simulink model "mfordmodel_v1"  (R2023a)
settings: Solver=ode45  StartTime=0.0  StopTime=10.0  RelTol=1e-3  EnableMultiTasking=on
undefined symbols (not defined in the file): ABV_RATIO_SW, AC_OFF_DLY, ACLOD, AUTO_TRNS_SW, BRAKE_DNDT_X, BZZRPM, BZZRPM_ALT, BZZTM, BZZTM_ALT, CMD_LITOFF, CMD_STABLE, CO_ST_ECT__A, COOL_BASE, DAS_BKDLY_A, DAS_CNT, DAS_CTDLY, DAS_LC_SW__A, DASCLP_5INH, DASCTL, DASMHYST, DASMPH, DEBYCP, DES_BASE, DPNEU_MUL, DSDRPM_DN_TC, DSDRPM_OFF, DSDRPM_UP_TC, EDF_DELAY, EDFHP, ETC_CL_TP, ETC_HP, GR_CM_CREEP, HCAM_ACT_CLP, HEDFHP, HEDFRPM, HICAM_PS, IAC_CAL_SW, IAC_ER_TM1, IAC_ER_TM2, IAC_ER_TM4, IAC_HI_LIM__A, IAC_ISFL_OBD, IAC_KAM_SW, IAC_LO_LIM__A, IAC_MON_TM, IAC_OT_REQ, IAC_RUN_TM, IAC_TP_OBD, IAC_TR_DAS, IAC_TST_DC, ID_DAS__A, ID_NOVS__A, IDVS_CH__A, IDVS_SL__A, IPSI_SW, IPSIDLY, IS_DRBASE__A, IS_DRBASE_A__A, IS_NUBASE__A, IS_NUBASE_A__A ... (+35)
libraries: simulink x2
(part 8 of 12)

== system mfordmodel_v1/iac_v04_001_001/normal_mode/iscflg_module/idle_rpm_controller/iscpsi_calc ==
  ml_tc_sw : Inport
  ml_iscpsi_sw : Inport  Port=2
  desmaf_pre : Inport  Port=3
  dsdrpm : Inport  Port=4
  rpmerr_a : Inport  Port=5
  iac_dlt_time : Inport  Port=6
  do_iscpsi_calc : TriggerPort  TriggerType=function-call  VariantControl=(inherit)
  Constant : Constant  Value=0.0
  Multiport Switch : MultiPortSwitch  Inputs=2
  Multiport Switch1 : MultiPortSwitch  Inputs=2
  Product : Product  Inputs=3  InputSameDT=on  RndMeth=Zero  SaturateOnIntegerOverflow=on  OutDataTypeStr=Inherit: Same as first input
  Product1 : Product  Inputs=*/  InputSameDT=on  RndMeth=Zero  SaturateOnIntegerOverflow=on  OutDataTypeStr=Inherit: Same as first input
  Product2 : Product  Inputs=*/  InputSameDT=on  RndMeth=Zero  SaturateOnIntegerOverflow=on  OutDataTypeStr=Inherit: Same as first input
  TC_OVER : Subsystem  mask(Constant){constant=TC_OVER}
      mask help: Constant Block. Will dispaly constant name and value on the icon of the block
      mask init:
      | if isletter(constant(1))
      |   const = evalin('base',constant);
      |   name = constant;
      | else
      |   const = str2num(constant);
      |   name = 'CONST';
      | end;
      mask Display: fprintf('%s = %.4f',name,const);
  TC_UNDER : Subsystem  mask(Constant){constant=TC_UNDER}
      mask help: Constant Block. Will dispaly constant name and value on the icon of the block
      mask init:
      | if isletter(constant(1))
      |   const = evalin('base',constant);
      |   name = constant;
      | else
      |   const = str2num(constant);
      |   name = 'CONST';
      | end;
      mask Display: fprintf('%s = %.4f',name,const);
  iscpsi : Outport
  wires:
  iac_dlt_time/1 -> Product2/1
  ml_tc_sw/1 -> Multiport Switch/1
  TC_OVER/1(Out) -> Multiport Switch/2
  TC_UNDER/1(Out) -> Multiport Switch/3
  Constant/1 -> Multiport Switch1/3
  ml_iscpsi_sw/1 -> Multiport Switch1/1
  Multiport Switch1/1 -> iscpsi/1  "iscpsi"
  Product/1 -> Multiport Switch1/2
  Multiport Switch/1 -> Product2/2
  Product2/1 -> Product/2
  rpmerr_a/1 -> Product/3
  dsdrpm/1 -> Product1/2
  desmaf_pre/1 -> Product1/1
  Product1/1 -> Product/1

== system mfordmodel_v1/iac_v04_001_001/normal_mode/iscflg_module/idle_rpm_controller/rpmerr_calc ==
  dsdrpm : Inport
  engine_speed : Inport  Port=2
  iac_dlt_time : Inport  Port=3
  ml_init_sw : Inport  Port=4
  do_rpmerr_calc : TriggerPort  TriggerType=function-call  VariantControl=(inherit)
  Constant3 : Constant  Value=0.0
  Constant4 : Constant  Value=0.0
  Multiport Switch4 : MultiPortSwitch  Inputs=2
  Multiport Switch5 : MultiPortSwitch  Inputs=2
  ROLAV_TC_DT_in : Subsystem  mask(Rolling Average - Time Constant){TAU=TCBPA}
      mask prompts: TAU "Time Constant"
      mask help: Rolling Average - Time Constant. This filter block is the first order approximation using a time constant. Inputs include the time constant (entered through this dialogue), old_ave which is the previous average value, new_value which is the new filter to filter toward, and the delta_time which is elapsed time over which to perform the filter equation.
      mask init:
      | if isletter(TAU(1))
      |   tc = evalin('base',TAU);
      |   name = TAU;
      | else
      |   tc = str2num(TAU);
      |   name = 'TC';
      | end;
      mask Display: fprintf('%s = %.4f',name,tc);
  Sum2 : Sum  Inputs=+-  InputSameDT=on  SaturateOnIntegerOverflow=on  OutDataTypeStr=Inherit: Same as first input
  Unit Delay : UnitDelay  SampleTime=-1
  rpmerr : Outport
  rpmerr_a : Outport  Port=2
  wires:
  ml_init_sw/1 -> Multiport Switch5/1, Multiport Switch4/1
  Multiport Switch5/1 -> Unit Delay/1, rpmerr_a/1  "rpmerr_a"
  Constant4/1 -> Multiport Switch5/3
  ROLAV_TC_DT_in/1(new_ave) -> Multiport Switch5/2  "rpmerr_a"
  Sum2/1 -> Multiport Switch4/2, ROLAV_TC_DT_in/1(new_value)  "rpmerr"
  Constant3/1 -> Multiport Switch4/3
  Multiport Switch4/1 -> rpmerr/1  "rpmerr"
  iac_dlt_time/1 -> ROLAV_TC_DT_in/3(delta_time)
  Unit Delay/1 -> ROLAV_TC_DT_in/2(old_ave)
  dsdrpm/1 -> Sum2/1
  engine_speed/1 -> Sum2/2

== system mfordmodel_v1/iac_v04_001_001/normal_mode/iscflg_module/iscflg_modes/1 ==
  note: Timer Control calls functions within the Time Calculator
      | after using the flags 'increment_flag' and 'decrement_flag'
      | to determine the direction of the timer.
  note: timer14/TIMER
  trig_time : Inport
  trig_reset : Inport  Port=2
  reset value : Inport  Port=3
  inc flag : Inport  Port=4
  dec flag : Inport  Port=5
  Event Triggers : Mux  Inputs=2
  Time Calculator : Subsystem
  Timer Control : Stateflow chart  TreatAsAtomicUnit=on
  timer : Outport
  wires:
  reset value/1 -> Time Calculator/5(reset_value)  "reset_value"
  trig_reset/1 -> Event Triggers/2  "trig_reset"
  trig_time/1 -> Event Triggers/1  "trig_timer"
  Event Triggers/1 -> Timer Control/Trigger
  Time Calculator/1(timer) -> timer/1  "timer"
  Timer Control/1(count_direction) -> Time Calculator/1(count_direction)  "count_direction"
  Timer Control/2(reset_flag) -> Time Calculator/2(reset_val)  "reset_flag"
  Timer Control/3(do_delta_time()) -> Time Calculator/3(do_delta_time)  "do_delta_time"
  Timer Control/4(do_timer()) -> Time Calculator/4(do_timer)  "do_timer"
  dec flag/1 -> Timer Control/2(decr_flag)  "decrement_flag"
  inc flag/1 -> Timer Control/1(incr_flag)  "increment_flag"

== system mfordmodel_v1/iac_v04_001_001/normal_mode/iscflg_module/iscflg_modes/2 ==
  note: Timer Control calls functions within the Time Calculator
      | after using the flags 'increment_flag' and 'decrement_flag'
      | to determine the direction of the timer.
  note: timer14/TIMER
  trig_time : Inport
  trig_reset : Inport  Port=2
  reset value : Inport  Port=3
  inc flag : Inport  Port=4
  dec flag : Inport  Port=5
  Event Triggers : Mux  Inputs=2
  Time Calculator : Subsystem
  Timer Control : Stateflow chart  TreatAsAtomicUnit=on
  timer : Outport
  wires:
  reset value/1 -> Time Calculator/5(reset_value)  "reset_value"
  trig_reset/1 -> Event Triggers/2  "trig_reset"
  trig_time/1 -> Event Triggers/1  "trig_timer"
  Event Triggers/1 -> Timer Control/Trigger
  Time Calculator/1(timer) -> timer/1  "timer"
  Timer Control/1(count_direction) -> Time Calculator/1(count_direction)  "count_direction"
  Timer Control/2(reset_flag) -> Time Calculator/2(reset_val)  "reset_flag"
  Timer Control/3(do_delta_time()) -> Time Calculator/3(do_delta_time)  "do_delta_time"
  Timer Control/4(do_timer()) -> Time Calculator/4(do_timer)  "do_timer"
  dec flag/1 -> Timer Control/2(decr_flag)  "decrement_flag"
  inc flag/1 -> Timer Control/1(incr_flag)  "increment_flag"

== system mfordmodel_v1/iac_v04_001_001/normal_mode/iscflg_module/preposition/idle_ppm_calc ==
  ml_mul_sw : Inport
  dsdrpm : Inport  Port=2
  engine_speed : Inport  Port=3
  ect : Inport  Port=4
  vspd : Inport  Port=5
  dstpbr : Inport  Port=6
  ratch : Inport  Port=7
  do_idle_ppm_calc : TriggerPort  TriggerType=function-call  VariantControl=(inherit)
  CONSTANT : Subsystem  mask(Constant){constant=DELHYS}
      mask help: Constant Block. Will dispaly constant name and value on the icon of the block
      mask init:
      | if isletter(constant(1))
      |   const = evalin('base',constant);
      |   name = constant;
      | else
      |   const = str2num(constant);
      |   name = 'CONST';
      | end;
      mask Display: fprintf('%s = %.4f',name,const);
  CONSTANT1 : Subsystem  mask(Constant){constant=DMAX_NEU_MOD}
      mask help: Constant Block. Will dispaly constant name and value on the icon of the block
      mask init:
      | if isletter(constant(1))
      |   const = evalin('base',constant);
      |   name = constant;
      | else
      |   const = str2num(constant);
      |   name = 'CONST';
      | end;
      mask Display: fprintf('%s = %.4f',name,const);
  CONSTANT2 : Subsystem  mask(Constant){constant=DASPTK}
      mask help: Constant Block. Will dispaly constant name and value on the icon of the block
      mask init:
      | if isletter(constant(1))
      |   const = evalin('base',constant);
      |   name = constant;
      | else
      |   const = str2num(constant);
      |   name = 'CONST';
      | end;
      mask Display: fprintf('%s = %.4f',name,const);
  Constant1 : Constant  Value=1.0
  Constant2 : Constant  Value=1.99
  Constant3 : Constant  Value=0.0
  FN814 : Subsystem  mask(2-D, piece-wise, linear interpolation){CAL_FUNC=FN814}
      mask prompts: CAL_FUNC "Calibration function name"
      mask help:
      | Performs piece-wise linear interpolation.
      |
      | Output is NOT extrapolated beyond the input range.  If the input value presented to the block lies outside the range specified in the block's parameter, then the value is treated as though it has the value of the nearest value in the range.
      mask init: same as mfordmodel_v1/iac_v04_001_001/activate_desired_rpm/rpm_calcs/lookup_2d
      mask Help:
      | Enter the name of the calibration function.
      | (e.g. EGM_VA_ECT_MULT)
      mask Display:
      | fprintf('%s',CAL_FUNC);
      | plot(calfunc.X,calfunc.Y,max_x*1.05,max_y*1.05,min_x,min_y);
  FN830__A : Subsystem  mask(2-D, piece-wise, linear interpolation){CAL_FUNC=FN830__A}
      mask prompts: CAL_FUNC "Calibration function name"
      mask help:
      | Performs piece-wise linear interpolation.
      |
      | Output is NOT extrapolated beyond the input range.  If the input value presented to the block lies outside the range specified in the block's parameter, then the value is treated as though it has the value of the nearest value in the range.
      mask init: same as mfordmodel_v1/iac_v04_001_001/activate_desired_rpm/rpm_calcs/lookup_2d
      mask Help:
      | Enter the name of the calibration function.
      | (e.g. EGM_VA_ECT_MULT)
      mask Display:
      | fprintf('%s',CAL_FUNC);
      | plot(calfunc.X,calfunc.Y,max_x*1.05,max_y*1.05,min_x,min_y);
  FN882A1 : Subsystem  mask(2-D, piece-wise, linear interpolation){CAL_FUNC=FN882A__A}
      mask prompts: CAL_FUNC "Calibration function name"
      mask help:
      | Performs piece-wise linear interpolation.
      |
      | Output is NOT extrapolated beyond the input range.  If the input value presented to the block lies outside the range specified in the block's parameter, then the value is treated as though it has the value of the nearest value in the range.
      mask init: same as mfordmodel_v1/iac_v04_001_001/activate_desired_rpm/rpm_calcs/lookup_2d
      mask Help:
      | Enter the name of the calibration function.
      | (e.g. EGM_VA_ECT_MULT)
      mask Display:
      | fprintf('%s',CAL_FUNC);
      | plot(calfunc.X,calfunc.Y,max_x*1.05,max_y*1.05,min_x,min_y);
  FN891 : Subsystem  mask(2-D, piece-wise, linear interpolation){CAL_FUNC=FN891}
      mask prompts: CAL_FUNC "Calibration function name"
      mask help:
      | Performs piece-wise linear interpolation.
      |
      | Output is NOT extrapolated beyond the input range.  If the input value presented to the block lies outside the range specified in the block's parameter, then the value is treated as though it has the value of the nearest value in the range.
      mask init: same as mfordmodel_v1/iac_v04_001_001/activate_desired_rpm/rpm_calcs/lookup_2d
      mask Help:
      | Enter the name of the calibration function.
      | (e.g. EGM_VA_ECT_MULT)
      mask Display:
      | fprintf('%s',CAL_FUNC);
      | plot(calfunc.X,calfunc.Y,max_x*1.05,max_y*1.05,min_x,min_y);
  MinMax : MinMax  Inputs=2  InputSameDT=on  SaturateOnIntegerOverflow=on
  MinMax1 : MinMax  Function=max  Inputs=2  InputSameDT=on  SaturateOnIntegerOverflow=on
  MinMax3 : MinMax  Inputs=2  InputSameDT=on  SaturateOnIntegerOverflow=on
  Multiport Switch4 : MultiPortSwitch  Inputs=2
  Product2 : Product  InputSameDT=on  RndMeth=Zero  SaturateOnIntegerOverflow=on  OutDataTypeStr=Inherit: Same as first input
  Product4 : Product  Inputs=****  InputSameDT=on  RndMeth=Zero  SaturateOnIntegerOverflow=on  OutDataTypeStr=Inherit: Same as first input
  Sum : Sum  Inputs=-+  InputSameDT=on  SaturateOnIntegerOverflow=on  OutDataTypeStr=Inherit: Same as first input
  Sum1 : Sum  Inputs=+-  InputSameDT=on  SaturateOnIntegerOverflow=on  OutDataTypeStr=Inherit: Same as first input
  Sum2 : Sum  InputSameDT=on  SaturateOnIntegerOverflow=on  OutDataTypeStr=Inherit: Same as first input
  Sum3 : Sum  InputSameDT=on  SaturateOnIntegerOverflow=on  OutDataTypeStr=Inherit: Same as first input
  idle_ppm : Outport
  wires:
  MinMax/1 -> idle_ppm/1  "idle_ppm"
  Constant3/1 -> MinMax1/1
  MinMax1/1 -> Product2/2  "idle_ppm_tmp"
  Sum1/1 -> MinMax1/2
  Constant2/1 -> MinMax3/2
  Product4/1 -> MinMax3/1  "dmax_nrm_tmp"
  MinMax3/1 -> MinMax/2  "dmax_fin_tmp"
  CONSTANT/1(Out) -> Sum2/2
  ratch/1 -> Sum2/1
  Sum/1 -> FN830__A/1(In1), [ml_n_dsdrpm]  "ml_n_dsdrpm"
  dsdrpm/1 -> Sum/1
  engine_speed/1 -> Sum/2
  dstpbr/1 -> Sum1/1
  Sum2/1 -> Sum1/2
  CONSTANT2/1(Out) -> Product2/1
  Product2/1 -> Sum3/2
  FN830__A/1(Out1) -> Sum3/1
  FN882A1/1(Out1) -> Product4/1
  ect/1 -> FN814/1(In1)
  ml_mul_sw/1 -> Multiport Switch4/1
  CONSTANT1/1(Out) -> Multiport Switch4/2
  Constant1/1 -> Multiport Switch4/3
  [ml_n_dsdrpm] -> FN882A1/1(In1)
  vspd/1 -> FN891/1(In1)
  FN891/1(Out1) -> Product4/2
  FN814/1(Out1) -> Product4/3
  Multiport Switch4/1 -> Product4/4  "dmax_neu_mul"
  Sum3/1 -> MinMax/1  "daspot_int_tmp"

== system mfordmodel_v1/iac_v04_001_001/iac_executive/fault_code_setting/TIMER_DT_in/Time Calculator/delta_time ==
  note: 'delta_time': the time interval
      | to be added to the timer for each cycle.
      | 'Gain' will adjust for second or millisecond timers.
  note: Timer direction is represented by
      | the multiplier 'count_direction'
      | 'count_direction' can be either -1, 0, or 1.
  count_direction : Inport
  count_direction1 : Inport  Port=2
  do_delta_time : TriggerPort  TriggerType=function-call  VariantControl=(inherit)
  Gain : Gain  Gain=unit_mul  SaturateOnIntegerOverflow=on  OutDataTypeStr=Inherit: Same as input  ParamDataTypeStr=Inherit: Same as input
  Product : Product  InputSameDT=on  RndMeth=Zero  SaturateOnIntegerOverflow=on  OutDataTypeStr=Inherit: Same as first input
  delta_time : Outport  InitialOutput=0
  wires:
  Gain/1 -> Product/2
  count_direction1/1 -> Gain/1  "delta_time"
  count_direction/1 -> Product/1  "count_direction"
  Product/1 -> delta_time/1  "delta_time"

== system mfordmodel_v1/iac_v04_001_001/iac_executive/fault_code_setting/TIMER_DT_in/Time Calculator/timer_calculation ==
  note: 'timer_calculation' takes the directional time increment 'delta_time'
      | and adds it to the previous timer value.  When the timer is reset,
      | all values are reset to 'reset_value'.
  note: 'Quantizer' switches the output
      |  to the appropriate resolution
      | based upon the top level
      |  dialog box selection.
  note: 'timer': cumulative
      | timer value
  note: 'init_value' provides the
      | initial value for the timer
  note: When 'reset_flag' is 1,
      |  'reset_value' is selected and
      | passed through the timer.
  reset_value : Inport
  reset_flag : Inport  Port=2
  delta_time : Inport  Port=3
  do_timer : TriggerPort  TriggerType=function-call  VariantControl=(inherit)
  Constant1 : Constant  Value=const_min
  Constant2 : Constant  Value=const_max
  Quantizer : Fcn  Expr=resolution*floor(u/resolution)
  Reset Switch : Switch  Threshold=0.5
  Sum : Sum  InputSameDT=on  SaturateOnIntegerOverflow=on  OutDataTypeStr=Inherit: Same as first input
  Terminator : Terminator
  Unit Delay : UnitDelay  InitialCondition=init_value  SampleTime=-1
  VAR SATURATION : Subsystem  mask(VARIABLE SATURATION){}
      mask help: This block will clip the input between the MIN and MAX values specified as inputs to the block. In addition a LIMIT_FLAG will be set to 1 if the input is currently being clipped.
      mask Display:
      | plot( [0.2 0.3 0.5 0.6], [0.2 0.2 0.8 0.8])
      | text(0.2, 0.05, 'min')
      | text(0.5, 0.95, 'max')
  lower bound = 0 : DeadZone  LowerValue=-inf  UpperValue=0.0
  timer : Outport  InitialOutput=0
  wires:
  VAR SATURATION/1(OUTPUT) -> Unit Delay/1, Quantizer/1
  VAR SATURATION/2(LIMIT_FLAG) -> Terminator/1
  Constant2/1 -> VAR SATURATION/1(MAX)
  Constant1/1 -> VAR SATURATION/3(MIN)
  lower bound = 0/1 -> VAR SATURATION/2(INPUT)
  Quantizer/1 -> timer/1  "timer"
  Unit Delay/1 -> Sum/2  "previous  timer value"
  Reset Switch/1 -> lower bound = 0/1
  reset_flag/1 -> Reset Switch/2  "reset_flag"
  reset_value/1 -> Reset Switch/1  "reset_value"
  delta_time/1 -> Sum/1  "delta_time"
  Sum/1 -> Reset Switch/3

== system mfordmodel_v1/iac_v04_001_001/iac_executive/misc_calcs/TIMER_DT_in/Time Calculator/delta_time ==
  note: 'delta_time': the time interval
      | to be added to the timer for each cycle.
      | 'Gain' will adjust for second or millisecond timers.
  note: Timer direction is represented by
      | the multiplier 'count_direction'
      | 'count_direction' can be either -1, 0, or 1.
  count_direction : Inport
  count_direction1 : Inport  Port=2
  do_delta_time : TriggerPort  TriggerType=function-call  VariantControl=(inherit)
  Gain : Gain  Gain=unit_mul  SaturateOnIntegerOverflow=on  OutDataTypeStr=Inherit: Same as input  ParamDataTypeStr=Inherit: Same as input
  Product : Product  InputSameDT=on  RndMeth=Zero  SaturateOnIntegerOverflow=on  OutDataTypeStr=Inherit: Same as first input
  delta_time : Outport  InitialOutput=0
  wires:
  Gain/1 -> Product/2
  count_direction1/1 -> Gain/1  "delta_time"
  count_direction/1 -> Product/1  "count_direction"
  Product/1 -> delta_time/1  "delta_time"

== system mfordmodel_v1/iac_v04_001_001/iac_executive/misc_calcs/TIMER_DT_in/Time Calculator/timer_calculation ==
  note: 'timer_calculation' takes the directional time increment 'delta_time'
      | and adds it to the previous timer value.  When the timer is reset,
      | all values are reset to 'reset_value'.
  note: 'Quantizer' switches the output
      |  to the appropriate resolution
      | based upon the top level
      |  dialog box selection.
  note: 'timer': cumulative
      | timer value
  note: 'init_value' provides the
      | initial value for the timer
  note: When 'reset_flag' is 1,
      |  'reset_value' is selected and
      | passed through the timer.
  reset_value : Inport
  reset_flag : Inport  Port=2
  delta_time : Inport  Port=3
  do_timer : TriggerPort  TriggerType=function-call  VariantControl=(inherit)
  Constant1 : Constant  Value=const_min
  Constant2 : Constant  Value=const_max
  Quantizer : Fcn  Expr=resolution*floor(u/resolution)
  Reset Switch : Switch  Threshold=0.5
  Sum : Sum  InputSameDT=on  SaturateOnIntegerOverflow=on  OutDataTypeStr=Inherit: Same as first input
  Terminator : Terminator
  Unit Delay : UnitDelay  InitialCondition=init_value  SampleTime=-1
  VAR SATURATION : Subsystem  mask(VARIABLE SATURATION){}
      mask help: This block will clip the input between the MIN and MAX values specified as inputs to the block. In addition a LIMIT_FLAG will be set to 1 if the input is currently being clipped.
      mask Display:
      | plot( [0.2 0.3 0.5 0.6], [0.2 0.2 0.8 0.8])
      | text(0.2, 0.05, 'min')
      | text(0.5, 0.95, 'max')
  lower bound = 0 : DeadZone  LowerValue=-inf  UpperValue=0.0
  timer : Outport  InitialOutput=0
  wires:
  VAR SATURATION/1(OUTPUT) -> Unit Delay/1, Quantizer/1
  VAR SATURATION/2(LIMIT_FLAG) -> Terminator/1
  Constant2/1 -> VAR SATURATION/1(MAX)
  Constant1/1 -> VAR SATURATION/3(MIN)
  lower bound = 0/1 -> VAR SATURATION/2(INPUT)
  Quantizer/1 -> timer/1  "timer"
  Unit Delay/1 -> Sum/2  "previous  timer value"
  Reset Switch/1 -> lower bound = 0/1
  reset_flag/1 -> Reset Switch/2  "reset_flag"
  reset_value/1 -> Reset Switch/1  "reset_value"
  delta_time/1 -> Sum/1  "delta_time"
  Sum/1 -> Reset Switch/3

== system mfordmodel_v1/iac_v04_001_001/iac_executive/mode_control/crank_mode/crank_calcs/lookup_2d FN818 ==
  In1 : Inport
  Look-Up Table1 : Lookup  InputValues=calfunc.X  Table=calfunc.Y
  Saturation1 : Saturate  UpperLimit=max_x  LowerLimit=min_x
  Out1 : Outport
  wires:
  In1/1 -> Saturation1/1
  Saturation1/1 -> Look-Up Table1/1
  Look-Up Table1/1 -> Out1/1

== system mfordmodel_v1/iac_v04_001_001/iac_executive/runup_flag_timer/TIMER_DT_in/Time Calculator/delta_time ==
  note: 'delta_time': the time interval
      | to be added to the timer for each cycle.
      | 'Gain' will adjust for second or millisecond timers.
  note: Timer direction is represented by
      | the multiplier 'count_direction'
      | 'count_direction' can be either -1, 0, or 1.
  count_direction : Inport
  count_direction1 : Inport  Port=2
  do_delta_time : TriggerPort  TriggerType=function-call  VariantControl=(inherit)
  Gain : Gain  Gain=unit_mul  SaturateOnIntegerOverflow=on  OutDataTypeStr=Inherit: Same as input  ParamDataTypeStr=Inherit: Same as input
  Product : Product  InputSameDT=on  RndMeth=Zero  SaturateOnIntegerOverflow=on  OutDataTypeStr=Inherit: Same as first input
  delta_time : Outport  InitialOutput=0
  wires:
  Gain/1 -> Product/2
  count_direction1/1 -> Gain/1  "delta_time"
  count_direction/1 -> Product/1  "count_direction"
  Product/1 -> delta_time/1  "delta_time"

== system mfordmodel_v1/iac_v04_001_001/iac_executive/runup_flag_timer/TIMER_DT_in/Time Calculator/timer_calculation ==
  note: 'timer_calculation' takes the directional time increment 'delta_time'
      | and adds it to the previous timer value.  When the timer is reset,
      | all values are reset to 'reset_value'.
  note: 'Quantizer' switches the output
      |  to the appropriate resolution
      | based upon the top level
      |  dialog box selection.
  note: 'timer': cumulative
      | timer value
  note: 'init_value' provides the
      | initial value for the timer
  note: When 'reset_flag' is 1,
      |  'reset_value' is selected and
      | passed through the timer.
  reset_value : Inport
  reset_flag : Inport  Port=2
  delta_time : Inport  Port=3
  do_timer : TriggerPort  TriggerType=function-call  VariantControl=(inherit)
  Constant1 : Constant  Value=const_min
  Constant2 : Constant  Value=const_max
  Quantizer : Fcn  Expr=resolution*floor(u/resolution)
  Reset Switch : Switch  Threshold=0.5
  Sum : Sum  InputSameDT=on  SaturateOnIntegerOverflow=on  OutDataTypeStr=Inherit: Same as first input
  Terminator : Terminator
  Unit Delay : UnitDelay  InitialCondition=init_value  SampleTime=-1
  VAR SATURATION : Subsystem  mask(VARIABLE SATURATION){}
      mask help: This block will clip the input between the MIN and MAX values specified as inputs to the block. In addition a LIMIT_FLAG will be set to 1 if the input is currently being clipped.
      mask Display:
      | plot( [0.2 0.3 0.5 0.6], [0.2 0.2 0.8 0.8])
      | text(0.2, 0.05, 'min')
      | text(0.5, 0.95, 'max')
  lower bound = 0 : DeadZone  LowerValue=-inf  UpperValue=0.0
  timer : Outport  InitialOutput=0
  wires:
  VAR SATURATION/1(OUTPUT) -> Unit Delay/1, Quantizer/1
  VAR SATURATION/2(LIMIT_FLAG) -> Terminator/1
  Constant2/1 -> VAR SATURATION/1(MAX)
  Constant1/1 -> VAR SATURATION/3(MIN)
  lower bound = 0/1 -> VAR SATURATION/2(INPUT)
  Quantizer/1 -> timer/1  "timer"
  Unit Delay/1 -> Sum/2  "previous  timer value"
  Reset Switch/1 -> lower bound = 0/1
  reset_flag/1 -> Reset Switch/2  "reset_flag"
  reset_value/1 -> Reset Switch/1  "reset_value"
  delta_time/1 -> Sum/1  "delta_time"
  Sum/1 -> Reset Switch/3

== system mfordmodel_v1/iac_v04_001_001/normal_mode/activate_feedforward/ac_ppm_tmr/Time Calculator/delta_time ==
  note: timer14/TIMER/Time Calculator/delta_time
  note: Timer direction is represented by
      | the multiplier 'count_direction'
      | 'count_direction' can be either -1, 0, or 1.
  note: 'delta_time': the time interval
      | to be added to the timer for each cycle.
      | 'Gain' will adjust for second or millisecond timers.
  count_direction : Inport
  do_delta_time : TriggerPort  TriggerType=function-call  VariantControl=(inherit)
  Gain : Gain  Gain=unit_mul  SaturateOnIntegerOverflow=on  OutDataTypeStr=Inherit: Same as input  ParamDataTypeStr=Inherit: Same as input
  Product : Product  InputSameDT=on  RndMeth=Zero  SaturateOnIntegerOverflow=on  OutDataTypeStr=Inherit: Same as first input
  Realtime Digital Clock : DigitalClock  SampleTime=-1
  Sum : Sum  Inputs=+-  InputSameDT=on  SaturateOnIntegerOverflow=on  OutDataTypeStr=Inherit: Same as first input
  Unit Delay1 : UnitDelay  SampleTime=-1
  delta_time : Outport  InitialOutput=0
  wires:
  Realtime Digital Clock/1 -> Sum/1, Unit Delay1/1  "timer"
  Gain/1 -> Product/2
  Sum/1 -> Gain/1
  Unit Delay1/1 -> Sum/2
  Product/1 -> delta_time/1  "delta_time"
  count_direction/1 -> Product/1  "count_direction"

== system mfordmodel_v1/iac_v04_001_001/normal_mode/activate_feedforward/ac_ppm_tmr/Time Calculator/timer_calculation ==
  note: When 'reset_flag' is 1,
      |  'reset_value' is selected and
      | passed through the timer.
  note: 'init_value' provides the
      | initial value for the timer
  note: 'timer': cumulative
      | timer value
  note: 'Quantizer' switches the output
      |  to the appropriate resolution
      | based upon the top level
      |  dialog box selection.
  note: 'timer_calculation' takes the directional time increment 'delta_time'
      | and adds it to the previous timer value.  When the timer is reset,
      | all values are reset to 'reset_value'.
  reset_value : Inport
  reset_flag : Inport  Port=2
  delta_time : Inport  Port=3
  do_timer : TriggerPort  TriggerType=function-call  VariantControl=(inherit)
  Constant1 : Constant  Value=const_min
  Constant2 : Constant  Value=const_max
  Quantizer5 : Fcn  Expr=resolution*floor(u/resolution)
  Reset Switch : Switch  Threshold=0.5
  Sum : Sum  InputSameDT=on  SaturateOnIntegerOverflow=on  OutDataTypeStr=Inherit: Same as first input
  Terminator : Terminator
  Unit Delay : UnitDelay  InitialCondition=init_value  SampleTime=-1
  VAR SATURATION : Subsystem  mask(VARIABLE SATURATION){}
      mask help: This block will clip the input between the MIN and MAX values specified as inputs to the block. In addition a LIMIT_FLAG will be set to 1 if the input is currently being clipped.
      mask Display:
      | plot( [0.2 0.3 0.5 0.6], [0.2 0.2 0.8 0.8])
      | text(0.2, 0.05, 'min')
      | text(0.5, 0.95, 'max')
  lower bound = 0 : DeadZone  LowerValue=-inf  UpperValue=0.0
  timer : Outport  InitialOutput=0
  wires:
  Quantizer5/1 -> timer/1  "timer"
  VAR SATURATION/1(OUTPUT) -> Quantizer5/1, Unit Delay/1
  Sum/1 -> Reset Switch/3
  delta_time/1 -> Sum/1  "delta_time"
  reset_value/1 -> Reset Switch/1  "reset_value"
  reset_flag/1 -> Reset Switch/2  "reset_flag"
  Reset Switch/1 -> lower bound = 0/1
  Unit Delay/1 -> Sum/2  "previous  timer value"
  lower bound = 0/1 -> VAR SATURATION/2(INPUT)
  Constant1/1 -> VAR SATURATION/3(MIN)
  Constant2/1 -> VAR SATURATION/1(MAX)
  VAR SATURATION/2(LIMIT_FLAG) -> Terminator/1

== system mfordmodel_v1/iac_v04_001_001/normal_mode/activate_kam/iac_kam_tmr/Time Calculator/delta_time ==
  note: timer14/TIMER/Time Calculator/delta_time
  note: Timer direction is represented by
      | the multiplier 'count_direction'
      | 'count_direction' can be either -1, 0, or 1.
  note: 'delta_time': the time interval
      | to be added to the timer for each cycle.
      | 'Gain' will adjust for second or millisecond timers.
  count_direction : Inport
  do_delta_time : TriggerPort  TriggerType=function-call  VariantControl=(inherit)
  Gain : Gain  Gain=unit_mul  SaturateOnIntegerOverflow=on  OutDataTypeStr=Inherit: Same as input  ParamDataTypeStr=Inherit: Same as input
  Product : Product  InputSameDT=on  RndMeth=Zero  SaturateOnIntegerOverflow=on  OutDataTypeStr=Inherit: Same as first input
  Realtime Digital Clock : DigitalClock  SampleTime=-1
  Sum : Sum  Inputs=+-  InputSameDT=on  SaturateOnIntegerOverflow=on  OutDataTypeStr=Inherit: Same as first input
  Unit Delay1 : UnitDelay  SampleTime=-1
  delta_time : Outport  InitialOutput=0
  wires:
  Realtime Digital Clock/1 -> Sum/1, Unit Delay1/1  "timer"
  Gain/1 -> Product/2
  Sum/1 -> Gain/1
  Unit Delay1/1 -> Sum/2
  Product/1 -> delta_time/1  "delta_time"
  count_direction/1 -> Product/1  "count_direction"

== system mfordmodel_v1/iac_v04_001_001/normal_mode/activate_kam/iac_kam_tmr/Time Calculator/timer_calculation ==
  note: When 'reset_flag' is 1,
      |  'reset_value' is selected and
      | passed through the timer.
  note: 'init_value' provides the
      | initial value for the timer
  note: 'timer': cumulative
      | timer value
  note: 'Quantizer' switches the output
      |  to the appropriate resolution
      | based upon the top level
      |  dialog box selection.
  note: 'timer_calculation' takes the directional time increment 'delta_time'
      | and adds it to the previous timer value.  When the timer is reset,
      | all values are reset to 'reset_value'.
  reset_value : Inport
  reset_flag : Inport  Port=2
  delta_time : Inport  Port=3
  do_timer : TriggerPort  TriggerType=function-call  VariantControl=(inherit)
  Constant1 : Constant  Value=const_min
  Constant2 : Constant  Value=const_max
  Quantizer5 : Fcn  Expr=resolution*floor(u/resolution)
  Reset Switch : Switch  Threshold=0.5
  Sum : Sum  InputSameDT=on  SaturateOnIntegerOverflow=on  OutDataTypeStr=Inherit: Same as first input
  Terminator : Terminator
  Unit Delay : UnitDelay  InitialCondition=init_value  SampleTime=-1
  VAR SATURATION : Subsystem  mask(VARIABLE SATURATION){}
      mask help: This block will clip the input between the MIN and MAX values specified as inputs to the block. In addition a LIMIT_FLAG will be set to 1 if the input is currently being clipped.
      mask Display:
      | plot( [0.2 0.3 0.5 0.6], [0.2 0.2 0.8 0.8])
      | text(0.2, 0.05, 'min')
      | text(0.5, 0.95, 'max')
  lower bound = 0 : DeadZone  LowerValue=-inf  UpperValue=0.0
  timer : Outport  InitialOutput=0
  wires:
  Quantizer5/1 -> timer/1  "timer"
  VAR SATURATION/1(OUTPUT) -> Quantizer5/1, Unit Delay/1
  Sum/1 -> Reset Switch/3
  delta_time/1 -> Sum/1  "delta_time"
  reset_value/1 -> Reset Switch/1  "reset_value"
  reset_flag/1 -> Reset Switch/2  "reset_flag"
  Reset Switch/1 -> lower bound = 0/1
  Unit Delay/1 -> Sum/2  "previous  timer value"
  lower bound = 0/1 -> VAR SATURATION/2(INPUT)
  Constant1/1 -> VAR SATURATION/3(MIN)
  Constant2/1 -> VAR SATURATION/1(MAX)
  VAR SATURATION/2(LIMIT_FLAG) -> Terminator/1

== system mfordmodel_v1/iac_v04_001_001/normal_mode/activate_normal_mode/ipsibr_clipping/ipsibr_clip/CONSTANT ==
  Constant : Constant  Value=const
  Out : Outport
  wires:
  Constant/1 -> Out/1

== system mfordmodel_v1/iac_v04_001_001/normal_mode/activate_normal_mode/ipsibr_clipping/ipsibr_clip/CONSTANT1 ==
  Constant : Constant  Value=const
  Out : Outport
  wires:
  Constant/1 -> Out/1

== system mfordmodel_v1/iac_v04_001_001/normal_mode/activate_normal_mode/ipsibr_clipping/ipsibr_clip/CONSTANT2 ==
  Constant : Constant  Value=const
  Out : Outport
  wires:
  Constant/1 -> Out/1

== system mfordmodel_v1/iac_v04_001_001/normal_mode/activate_normal_mode/ipsibr_clipping/ipsibr_clip/VAR_SATURATION ==
  note: IF INPUT <= MIN THEN SWITCH MIN ON
  note: IF INPUT >= MAX THEN SWITHMAX ON
  MAX : Inport
  INPUT : Inport  Port=2
  MIN : Inport  Port=3
  From : From
  From1 : From
  Goto : Goto
  Logical Operator : Logic  Operator=OR
  Relational Operator : RelationalOperator
  Relational Operator1 : RelationalOperator  Operator=<=
  Switch : Switch  Threshold=0.5
  Switch2 : Switch  Threshold=0.5
  SwitchMAX : Switch  Threshold=0.5
  OUTPUT : Outport
  LIMIT_FLAG : Outport  Port=2
  wires:
  MIN/1 -> Switch/1, Relational Operator1/2
  Switch/1 -> Switch2/3
  From1/1 -> SwitchMAX/3
  From/1 -> Switch/3
  INPUT/1 -> Goto/1, Relational Operator1/1, Relational Operator/1
  Switch2/1 -> OUTPUT/1
  SwitchMAX/1 -> Switch2/1
  MAX/1 -> SwitchMAX/1, Relational Operator/2
  Relational Operator/1 -> SwitchMAX/2, Switch2/2, Logical Operator/1
  Relational Operator1/1 -> Switch/2, Logical Operator/2
  Logical Operator/1 -> LIMIT_FLAG/1

== system mfordmodel_v1/iac_v04_001_001/normal_mode/activate_normal_mode/normal_mode_fault_codes/iac_er_tmr1/Time Calculator ==
  note: Calculates timer value.
      | Activated only when
      | counting up or down.
  note: Calculates time
      | between cycles.
      | Activated every cycle.
  note: Resets timer
      | to 'reset_value'
  note: Increment, hold,
      | or decrement
  note: Timer Control calls the counters 'delta_time' and 'timer_calculation'
      | after using the flags 'increment_flag' and 'decrement_flag'
      | to determine the direction of the timer.
  note: timer14/TIMER/Time Calculator
  count_direction : Inport
  reset_val : Inport  Port=2
  do_delta_time : Inport  Port=3
  do_timer : Inport  Port=4
  reset_value : Inport  Port=5
  From : From
  Goto : Goto
  delta_time : Subsystem  TreatAsAtomicUnit=on
  timer_calculation : Subsystem  TreatAsAtomicUnit=on
  timer : Outport
  wires:
  reset_value/1 -> timer_calculation/1(reset_value)  "reset_value"
  reset_val/1 -> timer_calculation/2(reset_flag)  "reset_flag"
  do_timer/1 -> timer_calculation/Trigger  "do_timer"
  From/1 -> timer_calculation/3(delta_time)  "delta_time"
  timer_calculation/1(timer) -> timer/1  "timer"
  count_direction/1 -> delta_time/1(count_direction)  "count_direction"
  delta_time/1(delta_time) -> Goto/1  "delta_time"
  do_delta_time/1 -> delta_time/Trigger  "do_delta_time"

== system mfordmodel_v1/iac_v04_001_001/normal_mode/activate_normal_mode/normal_mode_fault_codes/iac_er_tmr2/Time Calculator ==
  note: Calculates timer value.
      | Activated only when
      | counting up or down.
  note: Calculates time
      | between cycles.
      | Activated every cycle.
  note: Resets timer
      | to 'reset_value'
  note: Increment, hold,
      | or decrement
  note: Timer Control calls the counters 'delta_time' and 'timer_calculation'
      | after using the flags 'increment_flag' and 'decrement_flag'
      | to determine the direction of the timer.
  note: timer14/TIMER/Time Calculator
  count_direction : Inport
  reset_val : Inport  Port=2
  do_delta_time : Inport  Port=3
  do_timer : Inport  Port=4
  reset_value : Inport  Port=5
  From : From
  Goto : Goto
  delta_time : Subsystem  TreatAsAtomicUnit=on
  timer_calculation : Subsystem  TreatAsAtomicUnit=on
  timer : Outport
  wires:
  reset_value/1 -> timer_calculation/1(reset_value)  "reset_value"
  reset_val/1 -> timer_calculation/2(reset_flag)  "reset_flag"
  do_timer/1 -> timer_calculation/Trigger  "do_timer"
  From/1 -> timer_calculation/3(delta_time)  "delta_time"
  timer_calculation/1(timer) -> timer/1  "timer"
  count_direction/1 -> delta_time/1(count_direction)  "count_direction"
  delta_time/1(delta_time) -> Goto/1  "delta_time"
  do_delta_time/1 -> delta_time/Trigger  "do_delta_time"

== system mfordmodel_v1/iac_v04_001_001/normal_mode/activate_normal_mode/normal_mode_fault_codes/iac_mon_tmr/Time Calculator ==
  note: Calculates timer value.
      | Activated only when
      | counting up or down.
  note: Calculates time
      | between cycles.
      | Activated every cycle.
  note: Resets timer
      | to 'reset_value'
  note: Increment, hold,
      | or decrement
  note: Timer Control calls the counters 'delta_time' and 'timer_calculation'
      | after using the flags 'increment_flag' and 'decrement_flag'
      | to determine the direction of the timer.
  note: timer14/TIMER/Time Calculator
  count_direction : Inport
  reset_val : Inport  Port=2
  do_delta_time : Inport  Port=3
  do_timer : Inport  Port=4
  reset_value : Inport  Port=5
  From : From
  Goto : Goto
  delta_time : Subsystem  TreatAsAtomicUnit=on
  timer_calculation : Subsystem  TreatAsAtomicUnit=on
  timer : Outport
  wires:
  reset_value/1 -> timer_calculation/1(reset_value)  "reset_value"
  reset_val/1 -> timer_calculation/2(reset_flag)  "reset_flag"
  do_timer/1 -> timer_calculation/Trigger  "do_timer"
  From/1 -> timer_calculation/3(delta_time)  "delta_time"
  timer_calculation/1(timer) -> timer/1  "timer"
  count_direction/1 -> delta_time/1(count_direction)  "count_direction"
  delta_time/1(delta_time) -> Goto/1  "delta_time"
  do_delta_time/1 -> delta_time/Trigger  "do_delta_time"

== system mfordmodel_v1/iac_v04_001_001/normal_mode/activate_normal_mode/normal_mode_fault_codes/update_pids/  ==
  data : Inport
  ctrl : Inport  Port=2
  Terminator : Terminator
  Terminator1 : Terminator
  wires:
  ctrl/1 -> Terminator1/1
  data/1 -> Terminator/1

== system mfordmodel_v1/iac_v04_001_001/normal_mode/activate_normal_mode/normal_mode_fault_codes/update_pids/ 2 ==
  data : Inport
  ctrl : Inport  Port=2
  Terminator : Terminator
  Terminator1 : Terminator
  wires:
  ctrl/1 -> Terminator1/1
  data/1 -> Terminator/1

== system mfordmodel_v1/iac_v04_001_001/normal_mode/activate_normal_mode/normal_mode_fault_codes/update_pids/ 3 ==
  data : Inport
  ctrl : Inport  Port=2
  Terminator : Terminator
  Terminator1 : Terminator
  wires:
  ctrl/1 -> Terminator1/1
  data/1 -> Terminator/1

== system mfordmodel_v1/iac_v04_001_001/normal_mode/activate_normal_mode/output_flow_calc/desmaf_calc/CONSTANT ==
  Constant : Constant  Value=const
  Out : Outport
  wires:
  Constant/1 -> Out/1

== system mfordmodel_v1/iac_v04_001_001/normal_mode/activate_normal_mode/output_flow_calc/desmaf_calc/CONSTANT1 ==
  Constant : Constant  Value=const
  Out : Outport
  wires:
  Constant/1 -> Out/1

== system mfordmodel_v1/iac_v04_001_001/normal_mode/activate_normal_mode/output_flow_calc/desmaf_calc/CONSTANT2 ==
  Constant : Constant  Value=const
  Out : Outport
  wires:
  Constant/1 -> Out/1

== system mfordmodel_v1/iac_v04_001_001/normal_mode/activate_normal_mode/output_flow_calc/desmaf_calc/Clip ==
  In1 : Inport
  Saturation1 : Saturate  UpperLimit=max  LowerLimit=min
  Out1 : Outport
  wires:
  In1/1 -> Saturation1/1
  Saturation1/1 -> Out1/1

== system mfordmodel_v1/iac_v04_001_001/normal_mode/activate_normal_mode/output_flow_calc/desmaf_calc/lookup_2d FN035A ==
  In1 : Inport
  Look-Up Table1 : Lookup  InputValues=calfunc.X  Table=calfunc.Y
  Saturation1 : Saturate  UpperLimit=max_x  LowerLimit=min_x
  Out1 : Outport
  wires:
  In1/1 -> Saturation1/1
  Saturation1/1 -> Look-Up Table1/1
  Look-Up Table1/1 -> Out1/1

== system mfordmodel_v1/iac_v04_001_001/normal_mode/activate_normal_mode/output_flow_calc/desmaf_calc/lookup_2d FN059 ==
  In1 : Inport
  Look-Up Table1 : Lookup  InputValues=calfunc.X  Table=calfunc.Y
  Saturation1 : Saturate  UpperLimit=max_x  LowerLimit=min_x
  Out1 : Outport
  wires:
  In1/1 -> Saturation1/1
  Saturation1/1 -> Look-Up Table1/1
  Look-Up Table1/1 -> Out1/1

== system mfordmodel_v1/iac_v04_001_001/normal_mode/activate_normal_mode/output_flow_calc/desmaf_calc/lookup_2d FN818 ==
  In1 : Inport
  Look-Up Table1 : Lookup  InputValues=calfunc.X  Table=calfunc.Y
  Saturation1 : Saturate  UpperLimit=max_x  LowerLimit=min_x
  Out1 : Outport
  wires:
  In1/1 -> Saturation1/1
  Saturation1/1 -> Look-Up Table1/1
  Look-Up Table1/1 -> Out1/1

== system mfordmodel_v1/iac_v04_001_001/normal_mode/activate_normal_mode/output_flow_calc/desmaf_calc/lookup_2d FN819 ==
  In1 : Inport
  Look-Up Table1 : Lookup  InputValues=calfunc.X  Table=calfunc.Y
  Saturation1 : Saturate  UpperLimit=max_x  LowerLimit=min_x
  Out1 : Outport
  wires:
  In1/1 -> Saturation1/1
  Saturation1/1 -> Look-Up Table1/1
  Look-Up Table1/1 -> Out1/1

== system mfordmodel_v1/iac_v04_001_001/normal_mode/activate_normal_mode/output_flow_calc/desmaf_calc/lookup_2d FN890 ==
  In1 : Inport
  Look-Up Table1 : Lookup  InputValues=calfunc.X  Table=calfunc.Y
  Saturation1 : Saturate  UpperLimit=max_x  LowerLimit=min_x
  Out1 : Outport
  wires:
  In1/1 -> Saturation1/1
  Saturation1/1 -> Look-Up Table1/1
  Look-Up Table1/1 -> Out1/1

== system mfordmodel_v1/iac_v04_001_001/normal_mode/activate_normal_mode/output_flow_calc/desmaf_calc/lookup_3d ==
  X : Inport
  Y : Inport  Port=2
  Look-Up Table (2-D) : Lookup2D  RowIndex=caltable.Y  ColumnIndex=caltable.X  Table=caltable.Z
  Saturation1 : Saturate  UpperLimit=max_x  LowerLimit=min_x
  Saturation2 : Saturate  UpperLimit=max_y  LowerLimit=min_y
  Z : Outport
  wires:
  Look-Up Table (2-D)/1 -> Z/1  "z"
  Y/1 -> Saturation2/1
  X/1 -> Saturation1/1
  Saturation1/1 -> Look-Up Table (2-D)/2
  Saturation2/1 -> Look-Up Table (2-D)/1

== system mfordmodel_v1/iac_v04_001_001/normal_mode/iscflg_module/das_min_clip/functions/ROLAV_TC_DT_in1 ==
  note: Using the first two terms of the series expansion:
      |
      |                     x                     x2
      |                                e   =  1  +  x  +  --  + ......
      |                                           2!
      |
      |       Simplifying, the exponential "f" becomes:
      |
      |                  - (FK_TMR/TC)              1
      |           f  =  1  -  e                    =  1  -  -------------  =  . . .
      |                                                    (FK_TMR/TC)
      |                           e
      |
      |                              1                      1
      |          f  =  1  -  ---------------------------------  =    ------------------- .
      |                                  1 + (FK_TMR / TC)       1 + (TC / FK_TMR)
  note: - (FK_TMR/TC)
      |                                    f  =  1  -  e
      |
      |       Where "f" is called the filter constant in the difference equation:
      |
      |                    new_average = f * new_value + (1 - f) * old_average
  note: new_average = [ (sample_interval)/(sample_interval + time_constant) ] * (new_value - old_ave) + old_ave
  new_value : Inport
  old_ave : Inport  Port=2
  delta_time : Inport  Port=3
  Elementary Math : Math  Operator=reciprocal  SignedPower=on
  Product : Product  Inputs=3  InputSameDT=on  RndMeth=Zero  SaturateOnIntegerOverflow=on  OutDataTypeStr=Inherit: Same as first input
  Sum : Sum  Inputs=-+  InputSameDT=on  SaturateOnIntegerOverflow=on  OutDataTypeStr=Inherit: Same as first input
  Sum1 : Sum  InputSameDT=on  SaturateOnIntegerOverflow=on  OutDataTypeStr=Inherit: Same as first input
  Sum2 : Sum  InputSameDT=on  SaturateOnIntegerOverflow=on  OutDataTypeStr=Inherit: Same as first input
  Time Constant : Constant  Value=tc
  new_ave : Outport
  wires:
  Time Constant/1 -> Sum1/2
  Sum2/1 -> new_ave/1
  old_ave/1 -> Sum2/1, Sum/1
  Product/1 -> Sum2/2
  Sum/1 -> Product/1
  Elementary Math/1 -> Product/3
  Sum1/1 -> Elementary Math/1
  new_value/1 -> Sum/2
  delta_time/1 -> Product/2, Sum1/1

== system mfordmodel_v1/iac_v04_001_001/normal_mode/iscflg_module/das_min_clip/functions/ROLAV_TC_DT_in2 ==
  note: Using the first two terms of the series expansion:
      |
      |                     x                     x2
      |                                e   =  1  +  x  +  --  + ......
      |                                           2!
      |
      |       Simplifying, the exponential "f" becomes:
      |
      |                  - (FK_TMR/TC)              1
      |           f  =  1  -  e                    =  1  -  -------------  =  . . .
      |                                                    (FK_TMR/TC)
      |                           e
      |
      |                              1                      1
      |          f  =  1  -  ---------------------------------  =    ------------------- .
      |                                  1 + (FK_TMR / TC)       1 + (TC / FK_TMR)
  note: - (FK_TMR/TC)
      |                                    f  =  1  -  e
      |
      |       Where "f" is called the filter constant in the difference equation:
      |
      |                    new_average = f * new_value + (1 - f) * old_average
  note: new_average = [ (sample_interval)/(sample_interval + time_constant) ] * (new_value - old_ave) + old_ave
  new_value : Inport
  old_ave : Inport  Port=2
  delta_time : Inport  Port=3
  Elementary Math : Math  Operator=reciprocal  SignedPower=on
  Product : Product  Inputs=3  InputSameDT=on  RndMeth=Zero  SaturateOnIntegerOverflow=on  OutDataTypeStr=Inherit: Same as first input
  Sum : Sum  Inputs=-+  InputSameDT=on  SaturateOnIntegerOverflow=on  OutDataTypeStr=Inherit: Same as first input
  Sum1 : Sum  InputSameDT=on  SaturateOnIntegerOverflow=on  OutDataTypeStr=Inherit: Same as first input
  Sum2 : Sum  InputSameDT=on  SaturateOnIntegerOverflow=on  OutDataTypeStr=Inherit: Same as first input
  Time Constant : Constant  Value=tc
  new_ave : Outport
  wires:
  Time Constant/1 -> Sum1/2
  Sum2/1 -> new_ave/1
  old_ave/1 -> Sum2/1, Sum/1
  Product/1 -> Sum2/2
  Sum/1 -> Product/1
  Elementary Math/1 -> Product/3
  Sum1/1 -> Elementary Math/1
  new_value/1 -> Sum/2
  delta_time/1 -> Product/2, Sum1/1

== system mfordmodel_v1/iac_v04_001_001/normal_mode/iscflg_module/das_min_clip/functions/ROLAV_TC_DT_in3 ==
  note: Using the first two terms of the series expansion:
      |
      |                     x                     x2
      |                                e   =  1  +  x  +  --  + ......
      |                                           2!
      |
      |       Simplifying, the exponential "f" becomes:
      |
      |                  - (FK_TMR/TC)              1
      |           f  =  1  -  e                    =  1  -  -------------  =  . . .
      |                                                    (FK_TMR/TC)
      |                           e
      |
      |                              1                      1
      |          f  =  1  -  ---------------------------------  =    ------------------- .
      |                                  1 + (FK_TMR / TC)       1 + (TC / FK_TMR)
  note: - (FK_TMR/TC)
      |                                    f  =  1  -  e
      |
      |       Where "f" is called the filter constant in the difference equation:
      |
      |                    new_average = f * new_value + (1 - f) * old_average
  note: new_average = [ (sample_interval)/(sample_interval + time_constant) ] * (new_value - old_ave) + old_ave
  new_value : Inport
  old_ave : Inport  Port=2
  delta_time : Inport  Port=3
  Elementary Math : Math  Operator=reciprocal  SignedPower=on
  Product : Product  Inputs=3  InputSameDT=on  RndMeth=Zero  SaturateOnIntegerOverflow=on  OutDataTypeStr=Inherit: Same as first input
  Sum : Sum  Inputs=-+  InputSameDT=on  SaturateOnIntegerOverflow=on  OutDataTypeStr=Inherit: Same as first input
  Sum1 : Sum  InputSameDT=on  SaturateOnIntegerOverflow=on  OutDataTypeStr=Inherit: Same as first input
  Sum2 : Sum  InputSameDT=on  SaturateOnIntegerOverflow=on  OutDataTypeStr=Inherit: Same as first input
  Time Constant : Constant  Value=tc
  new_ave : Outport
  wires:
  Time Constant/1 -> Sum1/2
  Sum2/1 -> new_ave/1
  old_ave/1 -> Sum2/1, Sum/1
  Product/1 -> Sum2/2
  Sum/1 -> Product/1
  Elementary Math/1 -> Product/3
  Sum1/1 -> Elementary Math/1
  new_value/1 -> Sum/2
  delta_time/1 -> Product/2, Sum1/1

== system mfordmodel_v1/iac_v04_001_001/normal_mode/iscflg_module/das_min_clip/functions/ROLAV_TC_DT_in4 ==
  note: Using the first two terms of the series expansion:
      |
      |                     x                     x2
      |                                e   =  1  +  x  +  --  + ......
      |                                           2!
      |
      |       Simplifying, the exponential "f" becomes:
      |
      |                  - (FK_TMR/TC)              1
      |           f  =  1  -  e                    =  1  -  -------------  =  . . .
      |                                                    (FK_TMR/TC)
      |                           e
      |
      |                              1                      1
      |          f  =  1  -  ---------------------------------  =    ------------------- .
      |                                  1 + (FK_TMR / TC)       1 + (TC / FK_TMR)
  note: - (FK_TMR/TC)
      |                                    f  =  1  -  e
      |
      |       Where "f" is called the filter constant in the difference equation:
      |
      |                    new_average = f * new_value + (1 - f) * old_average
  note: new_average = [ (sample_interval)/(sample_interval + time_constant) ] * (new_value - old_ave) + old_ave
  new_value : Inport
  old_ave : Inport  Port=2
  delta_time : Inport  Port=3
  Elementary Math : Math  Operator=reciprocal  SignedPower=on
  Product : Product  Inputs=3  InputSameDT=on  RndMeth=Zero  SaturateOnIntegerOverflow=on  OutDataTypeStr=Inherit: Same as first input
  Sum : Sum  Inputs=-+  InputSameDT=on  SaturateOnIntegerOverflow=on  OutDataTypeStr=Inherit: Same as first input
  Sum1 : Sum  InputSameDT=on  SaturateOnIntegerOverflow=on  OutDataTypeStr=Inherit: Same as first input
  Sum2 : Sum  InputSameDT=on  SaturateOnIntegerOverflow=on  OutDataTypeStr=Inherit: Same as first input
  Time Constant : Constant  Value=tc
  new_ave : Outport
  wires:
  Time Constant/1 -> Sum1/2
  Sum2/1 -> new_ave/1
  old_ave/1 -> Sum2/1, Sum/1
  Product/1 -> Sum2/2
  Sum/1 -> Product/1
  Elementary Math/1 -> Product/3
  Sum1/1 -> Elementary Math/1
  new_value/1 -> Sum/2
  delta_time/1 -> Product/2, Sum1/1

== system mfordmodel_v1/iac_v04_001_001/normal_mode/iscflg_module/das_min_clip/functions/lookup_2d3 ==
  In1 : Inport
  Look-Up Table1 : Lookup  InputValues=calfunc.X  Table=calfunc.Y
  Saturation1 : Saturate  UpperLimit=max_x  LowerLimit=min_x
  Out1 : Outport
  wires:
  In1/1 -> Saturation1/1
  Saturation1/1 -> Look-Up Table1/1
  Look-Up Table1/1 -> Out1/1

== system mfordmodel_v1/iac_v04_001_001/normal_mode/iscflg_module/das_min_clip/functions/lookup_2d6 ==
  In1 : Inport
  Look-Up Table1 : Lookup  InputValues=calfunc.X  Table=calfunc.Y
  Saturation1 : Saturate  UpperLimit=max_x  LowerLimit=min_x
  Out1 : Outport
  wires:
  In1/1 -> Saturation1/1
  Saturation1/1 -> Look-Up Table1/1
  Look-Up Table1/1 -> Out1/1

== system mfordmodel_v1/iac_v04_001_001/normal_mode/iscflg_module/das_min_clip/functions/lookup_2d7 ==
  In1 : Inport
  Look-Up Table1 : Lookup  InputValues=calfunc.X  Table=calfunc.Y
  Saturation1 : Saturate  UpperLimit=max_x  LowerLimit=min_x
  Out1 : Outport
  wires:
  In1/1 -> Saturation1/1
  Saturation1/1 -> Look-Up Table1/1
  Look-Up Table1/1 -> Out1/1

== system mfordmodel_v1/iac_v04_001_001/normal_mode/iscflg_module/das_min_clip/functions/lookup_2d8 ==
  In1 : Inport
  Look-Up Table1 : Lookup  InputValues=calfunc.X  Table=calfunc.Y
  Saturation1 : Saturate  UpperLimit=max_x  LowerLimit=min_x
  Out1 : Outport
  wires:
  In1/1 -> Saturation1/1
  Saturation1/1 -> Look-Up Table1/1
  Look-Up Table1/1 -> Out1/1

== system mfordmodel_v1/iac_v04_001_001/normal_mode/iscflg_module/das_min_clip/functions/lookup_2d9 ==
  In1 : Inport
  Look-Up Table1 : Lookup  InputValues=calfunc.X  Table=calfunc.Y
  Saturation1 : Saturate  UpperLimit=max_x  LowerLimit=min_x
  Out1 : Outport
  wires:
  In1/1 -> Saturation1/1
  Saturation1/1 -> Look-Up Table1/1
  Look-Up Table1/1 -> Out1/1
